simulink library "GaitHandler"  (R2016b)
settings: Solver=VariableStepAuto  StartTime=0.0  StopTime=10.0  RelTol=1e-3
undefined symbols (not defined in the file or in its folder): ExokeletonState
libraries: lookUpTable x1, determinePhase x1, stateMachineHandler x1
settings Model: Creator=Nathan  LastModifiedBy=phil

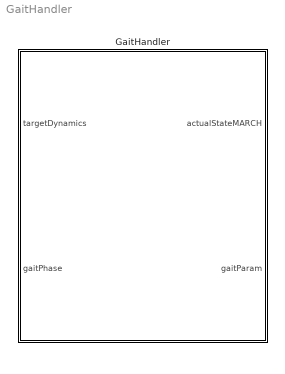
== system GaitHandler ==
  GaitHandler : Subsystem

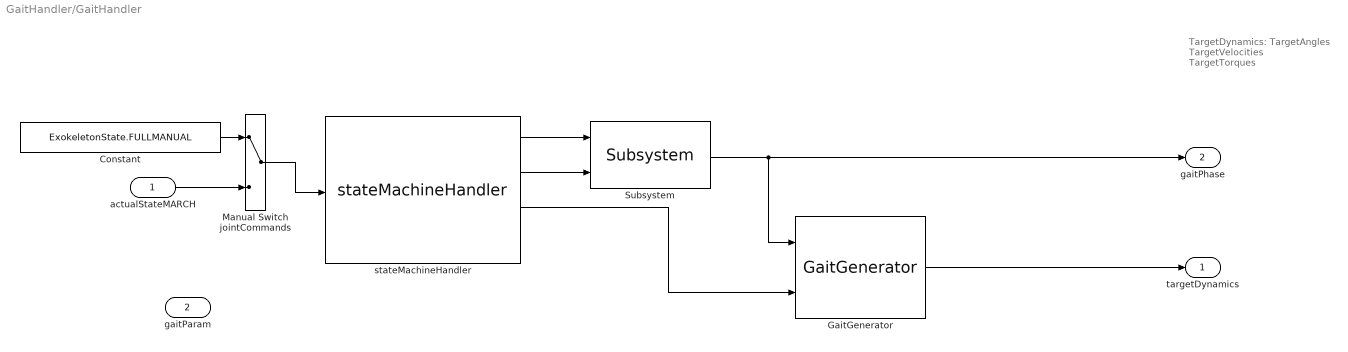
== system GaitHandler/GaitHandler ==
  note: TargetDynamics:
      | TargetAngles
      | TargetVelocities
      | TargetTorques
  actualStateMARCH : Inport
  gaitParam : Inport  Port=2
  Constant : Constant  Value=ExokeletonState.FULLMANUAL
  GaitGenerator : lookUpTable/GaitGenerator
  Manual Switch jointCommands : ManualSwitch
  Subsystem : determinePhase/stateMachineHandler/Subsystem
  stateMachineHandler : stateMachineHandler/stateMachineHandler
  targetDynamics : Outport  OutDataTypeStr=Bus: JointDynamics  PortDimensions=[1 4]  BusOutputAsStruct=on
  gaitPhase : Outport  Port=2
  wires:
  stateMachineHandler/2 -> Subsystem/2
  Constant/1 -> Manual Switch jointCommands/1
  Manual Switch jointCommands/1 -> stateMachineHandler/1
  actualStateMARCH/1 -> Manual Switch jointCommands/2
  stateMachineHandler/3 -> GaitGenerator/2
  GaitGenerator/1 -> targetDynamics/1
  stateMachineHandler/1 -> Subsystem/1
  Subsystem/1 -> gaitPhase/1, GaitGenerator/1
